simulink model "cl_ff01_sym"  (Simulink 8.1)
settings: Solver=ode3  StartTime=0.0  StopTime=100  FixedStep=T  RelTol=1e-3
values from neighbouring files (symbols this model uses):
  Gamma = [-4.33815; 0; 0]    [ss_engine_model.m]
  H = [0 0 -1]    [ss_engine_model.m]
  K1 = myacker(Phi, Gamma, z1)    [cl_fonp02.m]    (also in cl_fonp03.m = place(Phi, Gamma, z1))
  n = length(Phi)    [cl_fonp02.m]    (also in cl_fonp03.m; direct_design.m = order; sylvester.m = max(nA, nB) - 1)
  Phi = [0 0 -0.00237 ... (first row only)    [ss_engine_model.m]
  T = 1    [cd_plot1.m]    (also in cd_plot2.m; cl_ff01.m; cl_fonp02.m; cl_fonp03.m)
  x0 = [1; zeros(length(sysX.a) - 1, 1)]    [cl_ff01.m]    (also in cl_fonp02.m = rpm_lo*H; cl_fonp03.m = rpm_lo*H; lsim1.m = false)
undefined symbols (not defined in the file or in its folder): Lp
settings Model: Creator=jmahler  LastModifiedBy=jmahler
settings DataIOCC: SignalLoggingSaveFormat=Dataset
settings OptimizationCC: ExpressionDepthLimit=128
settings DebuggingCC: FcnCallInpInsideContextMsg=EnableAllAsError
settings GRTTargetCC: CombineOutputUpdateFcns=on  GRTInterface=off

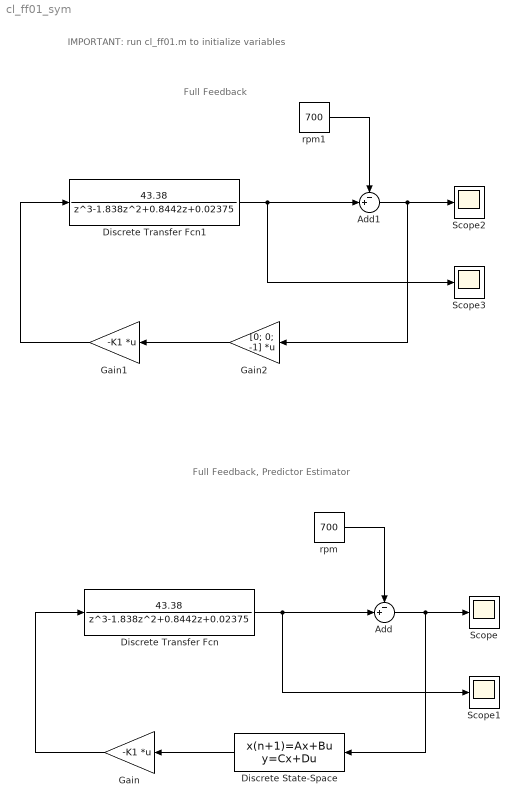
== system cl_ff01_sym ==
  note: Full Feedback
  note: Full Feedback, Predictor Estimator
  note: IMPORTANT: run cl_ff01.m to initialize variables
  Add : Sum  Inputs=-+|  SampleTime=T
  Add1 : Sum  Inputs=-+|  SampleTime=T
  Discrete Transfer Fcn : DiscreteTransferFcn  Numerator=[43.38]  Denominator=[1 -1.838 0.8442 0.02375]
  Discrete Transfer Fcn1 : DiscreteTransferFcn  Numerator=[43.38]  Denominator=[1 -1.838 0.8442 0.02375]
  Discrete State-Space : DiscreteStateSpace  A=(Phi - Gamma*K1 - Lp*H)  B=Lp  C=eye(n)  D=zeros(n,1)  X0=x0  SampleTime=T
  Gain : Gain  Gain=-K1  Multiplication=Matrix(K*u)  SampleTime=T
  Gain1 : Gain  Gain=-K1  Multiplication=Matrix(K*u)  SampleTime=T
  Gain2 : Gain  Gain=[0; 0; -1]  Multiplication=Matrix(K*u)  SampleTime=T
  Scope{,1..3} (4 alike) : Scope
      Scope2 settings: SaveName=ScopeData2
      Scope3 settings: SaveName=ScopeData3
  rpm : Constant  Value=700
  rpm1 : Constant  Value=700
  wires:
  Gain/1 -> Discrete Transfer Fcn/1
  Discrete Transfer Fcn/1 -> Scope1/1, Add/2
  rpm/1 -> Add/1
  Discrete State-Space/1 -> Gain/1
  Add/1 -> Discrete State-Space/1, Scope/1
  Gain1/1 -> Discrete Transfer Fcn1/1
  Discrete Transfer Fcn1/1 -> Scope3/1, Add1/2
  rpm1/1 -> Add1/1
  Add1/1 -> Gain2/1, Scope2/1
  Gain2/1 -> Gain1/1
